simulink model "Regelkreis_begrenzt"  (R2021a)
settings: Solver=VariableStepAuto  StartTime=0.0  StopTime=0.4  RelTol=1e-3
model workspace (MAT data in the model file):
  T1 = 0.01
  T2 = 0.1
  Tn = 0.1
  kp = 1
  u_max = 1.5
  u_min = -1.5
  v = 4
  w = 1
libraries: Regler x4
settings Model: Creator=Manoli  LastModifiedBy=Manoli

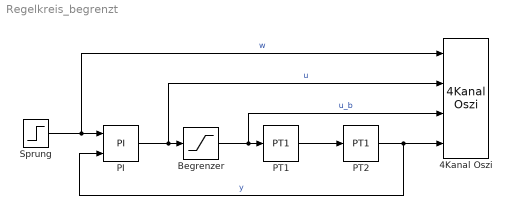
== system Regelkreis_begrenzt ==
  4Kanal Oszi : Regler/4Kanal Oszi  N=20000  k=[1 1 1 1]  y=[-5 5]  tmax=1
  Begrenzer : Saturate  UpperLimit=u_max  LowerLimit=u_min
  PI : Regler/PI  kp=kp  Tn=Tn
  PT1 : Regler/PT1  k=v  T1=T1
  PT2 : Regler/PT1  k=1  T1=T2
  Sprung : Step  Time=0.000001  After=w  SampleTime=0
  wires:
  PT1/1 -> PT2/1
  PT2/1 -> PI/2, 4Kanal Oszi/4  "y"
  Begrenzer/1 -> 4Kanal Oszi/3, PT1/1  "u_b"
  PI/1 -> 4Kanal Oszi/2, Begrenzer/1  "u"
  Sprung/1 -> PI/1, 4Kanal Oszi/1  "w"
